simulink model "MultiBody2024bfinal"  (R2024b)
settings: Solver=ode45  StartTime=0.0  StopTime=5  FixedStep=0.001  RelTol=1e-3  AbsTol=1e-3  EnableMultiTasking=on
InitFcn:
  | contact_damping = 1e4;
  | contact_stiffness = 1e6;
values from neighbouring files (symbols this model uses):
  Angle = [30 30 0]    [main_SuperTwistingSMC2.m]
  Height = -(1.9 + i)    (= -5.9)    [main_SuperTwistingSMC2.m]
  i = 4    [main_SuperTwistingSMC2.m]
  nt = n_t(i)    [main_SuperTwistingSMC2.m]
  TM = TMM(i)    [main_SuperTwistingSMC2.m]
  TotalWeight = TotalWeightmb(i)    [main_SuperTwistingSMC2.m]
undefined symbols (not defined in the file or in its folder): X, Y, Z
libraries: sm_lib x207, nesl_utility x73, sharedtransform x6, simulink_extras x4
(part 1 of 7)
settings Model: Creator=anaderi  LastModifiedBy=a.naderi
settings SolverCC: AutoScaleAbsTol=off  MaxZcPerStep=1
settings DataIOCC: LimitDataPoints=on  MaxDataPoints=10000
settings OptimizationCC: ReuseModelBlockBuffer=off  LifeSpan=inf
settings DebuggingCC: UnconnectedInputMsg=warning  UnconnectedOutputMsg=warning  UnconnectedLineMsg=warning  AllowSymbolicDim=off  SFUnexpectedBacktrackingDiag=warning  SFNoUnconditionalDefaultTransitionDiag=warning  SFExecutionAtInitializationDiag=none  ArithmeticOperatorsInVariantConditions=warning
settings ModelReferenceCC: EnableRefExpFcnMdlSchedulingChecks=on
settings SFSimCC: SimUseLocalCustomCode=off  CustomCodeUndefinedFunction=UseInterfaceOnly
settings RTWCC: RTWUseLocalCustomCode=off  GPUComputeCapability=3.5  DLArmComputeVersion=19.05
settings CodeAppCC: StateflowObjectComments=on
settings GRTTargetCC: TargetLangStandard=C89/C90 (ANSI)
settings ConfigComp: CovMetricSettings=dw  CovSaveCumulativeToWorkspaceVar=on  CovSaveSingleToWorkspaceVar=on  CovExternalEMLEnable=off  CovSFcnEnable=off
settings SimscapeCC: SimscapeLogType=all  SimscapeLogSimulationStatistics=on  SimscapeLogDataHistory=10000
settings ExplorerConfigSet: InternalSimMechanicsExplorerSettings="<ExplorerConfiguration><canonicalview>planar_xy</canonicalview><AnimationSetting><BasePlaybackSpeed>1.0</BasePlaybackSpeed><PlaybackSpeedFactor>1.0</PlaybackSpeedFactor></AnimationSetting><TilePanel><TileInfo><Tiles Columns=\"1\" Count=\"1\" Rows=\"1\"><Column Weight=\"1\"/><Row Weight=\"1\"/><Tile Height=\"1\" Width=\"1\" X=\"0\" Y=\"0\"/></Tiles></TileInfo><SceneInfo><SceneViewer><BGColor><R>1</R><G>1</G><B>1</B></BGColor><Camera><DoPerspective>off</DoPerspective><Position><X>-7.52643127180251614</X><Y>2.63618993258771184</Y><Z>6.23451341637808731</Z></Position><Center><X>-0.112830566017771972</X><Y>-0.116652157255869859</Y><Z>3.01253102664829608</Z></Center><Up><X>0.102173989792677611</X><Y>-0.627892603106608771</Y><Z>0.771564225955203575</Z></Up><ViewLimDist>1</ViewLimDist><YLim>1.72776258426052953</YLim><XLim>2.67975369164909827</XLim></Camera></SceneViewer></SceneInfo></TilePanel><MechEditorPanel><Cameras/><GfxPanelCameraMap/><VideoCreator><PlaybackSpeedRatio>1.0</PlaybackSpeedRatio><FrameRate>30</FrameRate><VideoFormat>Motion JPEG AVI</VideoFormat><FrameSize>auto</FrameSize></VideoCreator></MechEditorPanel></ExplorerConfiguration>"

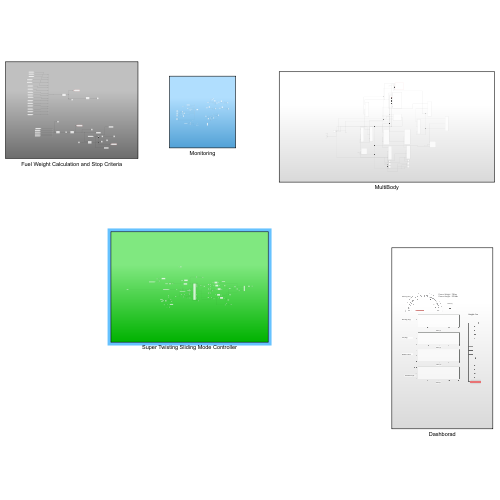
[thumbnail: Simulink's stored preview of the top-level diagram]
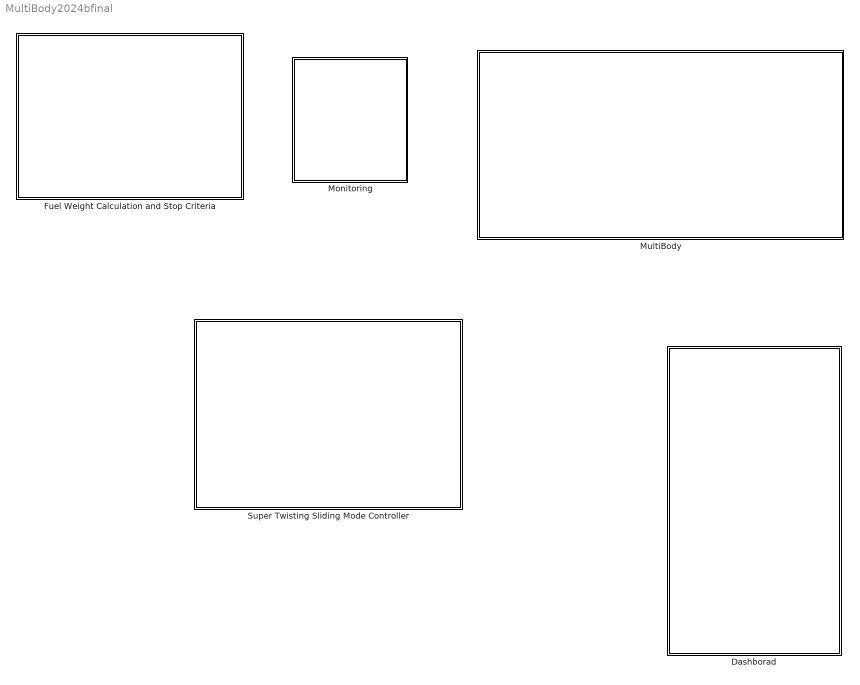
== system MultiBody2024bfinal ==
  Dashborad : Subsystem
  Fuel Weight Calculation and Stop Criteria : Subsystem
  Monitoring : Subsystem
  MultiBody : Subsystem
  Super Twisting Sliding Mode Controller : Subsystem

== system MultiBody2024bfinal/Dashborad ==
  note: Person Weight : 75 kg
      | Person Height : 170 cm
  note: Height: 3m
  note: Velocity (m/s)
  note: Time (s)
  note: Time (s)
  note: Bending (deg)
  note: Tilt (deg)
  note: Time (s)
  note: Rotation (deg)
  note: Time (s)
  note: Time (s)
  note: Disturbance (N)
  Dashboard Scope : DashboardScope  TimeSpan=2  Ymin=-50  Ymax=40  LegendPosition=InsideRight  ScaleAtStop=off
  Dashboard Scope1 : DashboardScope  TimeSpan=2  Ymin=-40  Ymax=30  LegendPosition=InsideRight  ScaleAtStop=off
  Dashboard Scope2 : DashboardScope  TimeSpan=2  Ymin=-180  Ymax=180  LegendPosition=InsideRight  ScaleAtStop=off
  Dashboard Scope3 : DashboardScope  TimeSpan=2  Ymin=0  Ymax=1100  LegendPosition=InsideRight  ScaleAtStop=off
  Display : DisplayBlock  LabelPosition=Hide  Transparency=1  Layout=Fill available space
  Half Gauge : SemiCircularGaugeBlock  LabelPosition=Hide  ScaleMax=12
  Vertical Gauge : CustomWebBlock  LabelPosition=Hide  ShowInitialText=on  Configuration="{\"components\":[{\"name\":\"LinearScaleComponent\",\"settings\":{\"bounds\":{\"max\":3,\"min\":0,\"tickInterval\":\"auto\"},\"internalTickHeightScaleFactor\":0.5,\"labelColor\":[0,0,0],\"labelFont\":{\"font\":\"Arial\",\"fontSize\":12},\"labelOffset\":0.05,\"labelTransparency\":1,\"needleImage\":{\"size\":[21,75],\"src\":\"data:image\\/svg+xml;base64,PHN2ZyB4bWxucz0iaHR0cDovL3d3dy53My5vcmcvMjAwMC9zdmciIHhtbG5zOnhsaW5rPSJodHRwOi8vd3d3LnczLm9yZy8xOTk5L3hsaW5rIiB2aWV3Qm94PSIwIDAgMjEgNzUiPjxkZWZzPjxzdHlsZT4uY2xzLTF7ZmlsbDpub25lO30uY2xzLTJ7aXNvbGF0aW9uOmlzb2xhdGU7fS5jbHMtM3tjbGlwLXBhdGg6dXJsKCNjbGlwLXBhdGgpO30uY2xzLTR7b3BhY2l0eTowLjM7bWl4LWJsZW5kLW1vZGU6bXVsdGlwbHk7fS5jbHMtNXtmaWxsOiNlYjI2Mjk7fTwvc3R5bGU+PGNsaXBQYXRoIGlkPSJjbGlwLXBhdGgiIHRyYW5zZm9y ...(+1928 chars)\",\"srcOrientation\":\"horizontal\"},\"needleOffset\":[0.007413509060955519,0],\"needleSize\":{\"height\":0.11955094537815127,\"width\":0.7589285714285714},\"position\":[0.015811846038863975,0.0696875,0.79984375,0.9641489162929746],\"referencePoint\":\"auto\",\"scaleColors\":[],\"scaleColorsSize\":0.2,\"scaleDirection\":\"BT\",\"showLabels\":1,\"showMinorTicks\":0,\"showSpanLine\":1,\"showTicks\":1,\"tickColor\":[0,0,0],\"tickTransparency\":1,\"valueBarColor\":[23,89,176],\"valueBarOffset\":-1,\"valueBarSize\":0,\"valueBarTransparency\":1}},{\"name\":\"BackgroundImageComponent\",\"settings\":{\"image\":{\"size\":[380,101],\"src\":\"data:image\\/svg+xml;base64,PHN2ZyBpZD0iZnJhbWUiIHhtbG5zPSJodHRwOi8vd3d3LnczLm9yZy8yMDAwL3N2ZyIgeG1sbnM6eGxpbms9Imh0dHA6Ly93d3cudzMub3JnLzE5OTkveGxpbmsiIHZpZXdCb3g9IjAgMCAzODAgMTAxIj48ZGVmcz48c3R5bGU+LmNscy0xe2ZpbGw6IzAwMmI0Mjt9LmNscy0ye2ZpbGw6IzQyNzA4Mjt9LmNscy0ze2ZpbGw6dXJsKCNyYWRpYWwtZ3JhZGllbnQpO308L3N0eWxlPjxyYWRpYWxHcmFkaWVudCBpZD0icmFkaWFsLWdyYWRpZW50IiBjeD0iMTkwIiBjeT0iNTAuNSIgcj0iMjY5LjIxIiBncmFkaWVudFVuaXRzPSJ1c2VyU3BhY2VPblVzZSI+PHN0b3Agb2Zmc2V0PSIwLjAxIiBzdG9wLWNvbG9yPSIjM2U0ZjU4Ii8+PHN0b3Agb2Zmc2V0PSIwLjA2IiBzdG9wLWNvbG9yPSIjNDQ1NzYxIi8+PHN0b3Agb2Zmc2V0PSIwLjE1IiBzdG9wLWNvbG9yPSIjNTU2YTc2Ii8+PHN0b3Agb2Zmc2V0PSIwLjI1IiBzdG9wLWNvbG9yPSIjNmQ4ODk1Ii8+PHN0b3Agb2Zmc2V0PSIwLjM4IiBzdG9wLWNvbG9yPSIjOGZiMmMzIi8+PHN0b3Agb2Zmc2V0PSIwLjUyIiBzdG9wLWNvbG9yPSIjYjZlNGZhIi8+PHN0b3Agb2Zmc2V0PSIxIiBzdG9wLWNvbG9yPSIjMTU0NjU3Ii8+PC9yYWRpYWxHcmFkaWVudD48L2RlZnM+PGcgaWQ9IkxheWVyXzIiIGRhdGEtbmFtZT0iTGF5ZXIgMiI+PGcgaWQ9IkxheWVyXzEtMiIgZGF0YS1uYW1lPSJMYXllciAxLTIiPjxyZWN0IGlkPSJyZWN0MTAzNiIgY2xhc3M9ImNscy0xIiB4PSIxMSIgeT0iMTEiIHdpZHRoPSIzNTgiIGhlaWdodD0iNzkiLz48cGF0aCBpZD0icGF0aDEwMzgiIGNsYXNzPSJjbHMtMiIgZD0iTTgsOFY5M0gzNzJWOFpNMzY5LDkwSDExVjExSDM2OVoiLz48cGF0aCBpZD0icGF0aDEwNDAiIGNsYXNzPSJjbHMtMyIgZD0iTTAsMFYxMDFIMzgwVjBaTTM3Miw5M0g4VjhIMzcyWiIvPjwvZz48L2c+PC9zdmc+\",\"srcOrientation\":\"horizontal\"},\"position\":[0,0,1,1],\"scaleMode\":\"0\"}},{\"name\":\"ForegroundImageComponent\",\"settings\":{\"image\":{\"size\":[0,0],\"src\":\"default\",\"srcOrientation\":[]},\"isForeground\":1,\"position\":[0,0,1,1],\"scaleMode\":\"0\"}}],\"settings\":{\"BindingType\":\"signal\",\"backgroundColor\":[0,0,0,\"1\"],\"backgroundOffset\":0,\"backgroundOpacity\":0,\"fixedAspectRatio\":\"off\",\"orientation\":\"vertical\",\"showBackgroundColor\":false,\"value\":0,\"version\":\"R2022b\"},\"type\":\"LinearGauge\"}"  CustomBackgroundColor="{\"color\":[1,1,1],\"show\":true}"

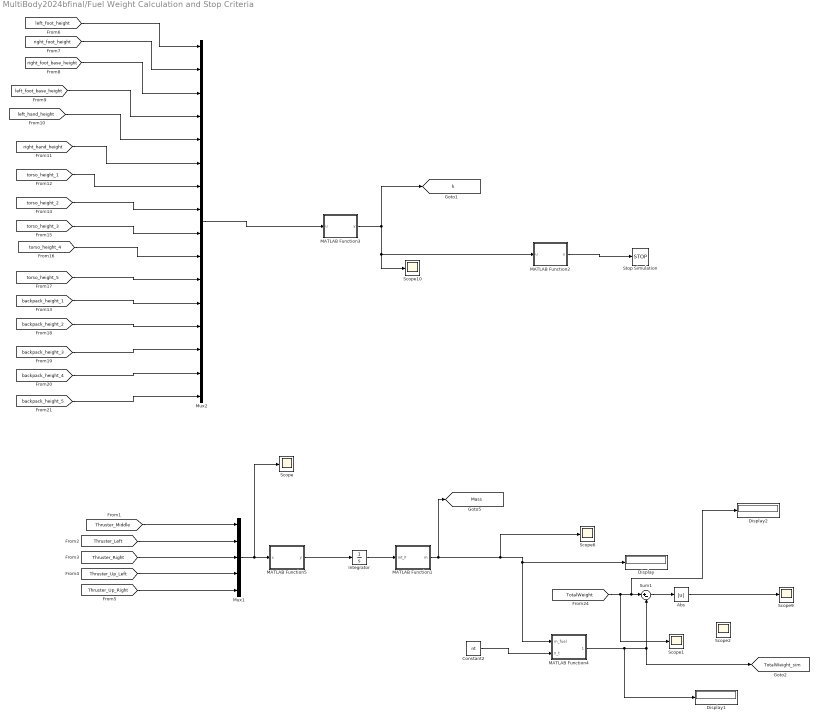
== system MultiBody2024bfinal/Fuel Weight Calculation and Stop Criteria ==
  Abs : Abs  SaturateOnIntegerOverflow=off
  Constant2 : Constant  Value=nt
  Display : Display
  Display1 : Display
  Display2 : Display
  Integrator : Integrator
  MATLAB Function1 : MATLAB Function  TreatAsAtomicUnit=on
  MATLAB Function2 : MATLAB Function  TreatAsAtomicUnit=on
  MATLAB Function3 : MATLAB Function  TreatAsAtomicUnit=on
  MATLAB Function4 : MATLAB Function  TreatAsAtomicUnit=on
  MATLAB Function5 : MATLAB Function  TreatAsAtomicUnit=on
  Mux1 : Mux  Inputs=5
  Mux2 : Mux  Inputs=16
  Scope{,1..2,6,9..10} (6 alike) : Scope
  Stop Simulation : Stop
  Sum1 : Sum  Inputs=|+-
  tag scope: Mass=global, TotalWeight_sim=global, h=global
  wires:
  [torso_height_2] -> Mux2/8
  MATLAB Function4/1(m_total) -> Display1/1, Sum1/2, [TotalWeight_sim]
  MATLAB Function1/1(m) -> Scope6/1, MATLAB Function4/1(m_fuel), Display/1, [Mass]
  MATLAB Function5/1(y) -> Integrator/1
  [backpack_height_2] -> Mux2/13
  [right_foot_height] -> Mux2/2
  [backpack_height_1] -> Mux2/12
  [left_foot_base_height] -> Mux2/4
  [backpack_height_4] -> Mux2/15
  Sum1/1 -> Abs/1
  Mux1/1 -> Scope/1, MATLAB Function5/1(x)
  Mux2/1 -> MATLAB Function3/1(u)
  [right_hand_height] -> Mux2/6
  [backpack_height_5] -> Mux2/16
  [torso_height_3] -> Mux2/9
  [torso_height_5] -> Mux2/11
  [Thruster_Right] -> Mux1/3
  [left_hand_height] -> Mux2/5
  [torso_height_4] -> Mux2/10
  [backpack_height_3] -> Mux2/14
  MATLAB Function2/1(y) -> Stop Simulation/1
  [left_foot_height] -> Mux2/1
  [Thruster_Up_Left] -> Mux1/4
  MATLAB Function3/1(y) -> MATLAB Function2/1(u), Scope10/1, [h]
  [Thruster_Middle] -> Mux1/1
  [right_foot_base_height] -> Mux2/3
  [torso_height_1] -> Mux2/7
  [Thruster_Up_Right] -> Mux1/5
  Abs/1 -> Scope9/1
  [Thruster_Left] -> Mux1/2
  Constant2/1 -> MATLAB Function4/2(n_t)
  Integrator/1 -> MATLAB Function1/1(int_F)
  [TotalWeight] -> Scope1/1, Display2/1, Sum1/1

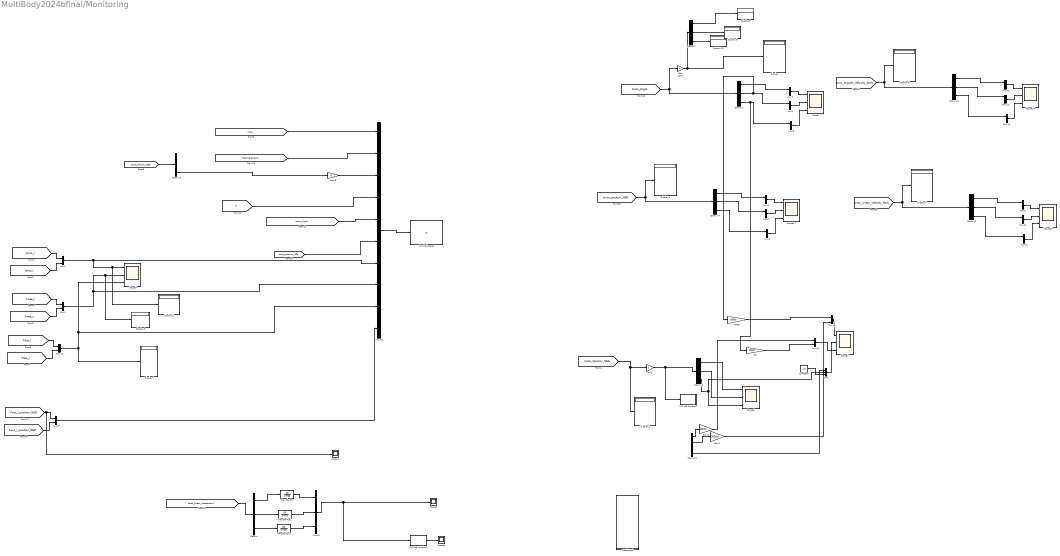
== system MultiBody2024bfinal/Monitoring ==
  Constant : Constant  Value=4.8
  Dashborad : Subsystem
  Demux{,1..4,6..8} (8 alike) : Demux  Outputs=3
  Demux5 : Demux
  Display{,1..10} (11 alike) : Display
  Gain : Gain  Gain=180/pi
  Gain1 : Gain  Gain=180/pi
  Gain6 : Gain  Gain=180/pi
  Gain8 : Gain  Gain=-1
  MATLAB Function : MATLAB Function  TreatAsAtomicUnit=on
  MATLAB Function1 : MATLAB Function  TreatAsAtomicUnit=on
  Mux : Mux  Inputs=3
  Mux{1..15,17,19..20} (18 alike) : Mux  Inputs=2
  Mux16 : Mux  Inputs=10
  Mux18 : Mux  Inputs=3
  Phi : Gain  Gain=180/pi
  Phi2 : Gain
  Scope{,1..3,17,19..20} (7 alike) : Scope  NumInputPorts=3
  Scope4 : Scope
  Scope5 : Scope
  Scope6 : Scope
  Theta : Gain  Gain=180/pi
  To Workspace : ToWorkspace  VariableName=x  SampleTime=-1
      settings: Save2DSignal=2-D array (concatenate along first dimension)
  Transfer Fcn : TransferFcn  Numerator=[50]  Denominator=[1 50]
  Transfer Fcn1 : TransferFcn  Numerator=[50]  Denominator=[1 50]
  Transfer Fcn2 : TransferFcn  Numerator=[50]  Denominator=[1 50]
  wires:
  [torso_Angle] -> Demux2/1, Gain/1
  [torso_position_NED] -> Demux4/1, Display2/1
  Mux7/1 -> Scope17/2
  Demux4/2 -> Mux7/1
  [torso_Linear_Velocity_Body] -> Display4/1, Demux6/1
  Mux4/1 -> Scope/2
  Demux6/1 -> Mux9/1
  Demux2/2 -> Theta/1, Mux4/1
  [torso_Angular_Velocity_Body] -> Demux8/1, Display6/1
  Demux6/2 -> Mux10/1
  Mux10/1 -> Scope19/2
  Mux6/1 -> Scope17/1
  Mux9/1 -> Scope19/1
  Mux11/1 -> Scope19/3
  Mux12/1 -> Scope20/2
  Mux8/1 -> Scope17/3
  Mux14/1 -> Scope20/1
  Mux5/1 -> Scope/3
  Mux3/1 -> Scope/1
  Demux8/1 -> Mux14/1
  Demux2/3 -> Phi/1, Mux5/1
  Demux4/1 -> Mux6/1
  Demux2/1 -> Mux3/1
  Demux8/3 -> Mux13/1
  Demux8/2 -> Mux12/1
  Demux6/3 -> Mux11/1
  Mux13/1 -> Scope20/3
  Demux4/3 -> Mux8/1
  Theta/1 -> Mux19/1
  [torso_Velocity_NED] -> Display1/1, Phi2/1
  Demux1/3 -> Mux/2, Scope2/3
  Phi/1 -> Mux20/2
  Gain/1 -> Demux7/1, Display/1
  Constant/1 -> Mux/3
  Mux/1 -> Scope1/2
  Demux1/1 -> Scope2/1
  Demux1/2 -> Scope2/2
  Phi2/1 -> Demux1/1, MATLAB Function/1(u)
  [torso_r] -> Mux1/1
  [torso_l] -> Mux1/2
  [knee_r] -> Mux2/2
  [knee_l] -> Mux2/1
  [Tibia_l] -> Mux15/1
  [Tibia_r] -> Mux15/2
  Mux2/1 -> Mux16/8, Display5/1, Scope3/2
  [torso_Velocity_NED] -> Demux3/1
  Demux3/3 -> Gain8/1
  [torso_Angle] -> Mux16/5
  Mux16/1 -> To Workspace/1
  [TotalWeight_sim] -> Mux16/2
  [torso_position_NED] -> Mux16/6
  Gain8/1 -> Mux16/3
  [h] -> Mux16/4
  [Mass] -> Mux16/1
  Mux1/1 -> Mux16/7, Display3/1, Scope3/1
  Mux15/1 -> Mux16/9, Scope3/3, Display7/1
  [Foot_r_position_NED] -> Mux17/2
  [Foot_l_position_NED] -> Scope4/1, Mux17/1
  Mux17/1 -> Mux16/10
  Mux18/1 -> MATLAB Function1/1(u), Scope5/1
  [torso_Linear_Acceleration] -> Demux/1
  Demux/1 -> Transfer Fcn/1
  Transfer Fcn/1 -> Mux18/1
  Demux/2 -> Transfer Fcn1/1
  Transfer Fcn1/1 -> Mux18/2
  Demux/3 -> Transfer Fcn2/1
  Transfer Fcn2/1 -> Mux18/3
  MATLAB Function1/1(y) -> Scope6/1
  Demux5/2 -> Gain1/1
  ? -> Demux5/1
  Demux5/1 -> Gain6/1
  Gain1/1 -> Mux19/2
  Mux19/1 -> Scope1/1
  Gain6/1 -> Mux20/1
  Mux20/1 -> Scope1/3
  Demux5/4 -> Mux/1
  Demux7/1 -> Display8/1
  Demux7/2 -> Display9/1
  Demux7/3 -> Display10/1

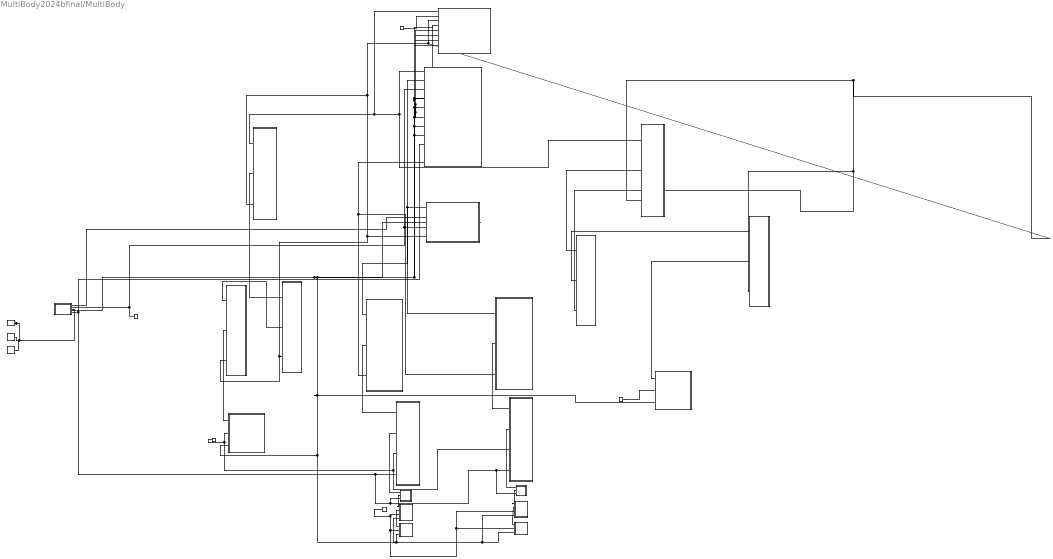
== system MultiBody2024bfinal/MultiBody ==
  Connection Label{1..5} (5 alike) : ConnectionLabel  Label=Ground
  Femur_r : Subsystem
      mask Display: image('$imagefile');
  Femur_r1 : Subsystem
      mask Display: image('$imagefile'); % Use "Edit Image" on toolstrip to change.
  Femur_r10 : Subsystem
      mask Display: image('$imagefile'); % Use "Edit Image" on toolstrip to change.
  Femur_r11 : Subsystem
      mask Display: image('$imagefile'); % Use "Edit Image" on toolstrip to change.
  Femur_r12 : Subsystem
      mask Display: image('$imagefile'); % Use "Edit Image" on toolstrip to change.
  Femur_r13 : Subsystem
      mask Display: image('$imagefile'); % Use "Edit Image" on toolstrip to change.
  Femur_r14 : Subsystem
      mask Display: image('$imagefile'); % Use "Edit Image" on toolstrip to change.
  Femur_r15 : Subsystem
      mask Display: image('$imagefile'); % Use "Edit Image" on toolstrip to change.
  Femur_r2 : Subsystem
      mask Display: image('$imagefile'); % Use "Edit Image" on toolstrip to change.
  Femur_r3 : Subsystem
      mask Display: image('$imagefile'); % Use "Edit Image" on toolstrip to change.
  Femur_r4 : Subsystem
      mask Display: image('$imagefile'); % Use "Edit Image" on toolstrip to change.
  Femur_r5 : Subsystem
      mask Display: image('$imagefile'); % Use "Edit Image" on toolstrip to change.
  Femur_r6 : Subsystem
      mask Display: image('$imagefile'); % Use "Edit Image" on toolstrip to change.
  Femur_r7 : Subsystem
      mask Display: image('$imagefile'); % Use "Edit Image" on toolstrip to change.
  Femur_r8 : Subsystem
      mask Display: image('$imagefile'); % Use "Edit Image" on toolstrip to change.
  Femur_r9 : Subsystem
      mask Display: image('$imagefile'); % Use "Edit Image" on toolstrip to change.
  Grpund : Subsystem
  Mechanism Configuration : sm_lib/Utilities/Mechanism Configuration  UniformGravity=Constant  GravityVector=[0 0 -9.80665]  GravityVectorUnits=m/s^2  LinearizationDelta=0.001  JointModeTransitionNonlinearIterations=2
  Pelvos : Subsystem
      mask Display: image('$imagefile'); % Use "Edit Image" on toolstrip to change.
  Solver Configuration : nesl_utility/Solver Configuration  PhysicalDomain=network_engine_domain  SubClassName=solver  LeftPortType=input  RightPortType=generic  Tones=[]  Harmonics=[]  SimulateNoise=off  Profile=off  UseLocalSampling=off  EnableSwitchedLinearOptims=on  FrequencyDomain=off  UseCCode=off  RelTol=0.001  AbsTol=1e-06  MinStep=1e-09  ToWorkspace=off  RevertToSquareIcSolve=off  NumHomotopyIterations=100  PhasorMode=off  PhasorModeNumHarmonics=1  ConsistencySolver=NEWTON_FTOL  IndexReductionMethod=DerivativeReplacement  DoDC=off  ResidualTolerance=1e-09  ConsistencyTolSource=GLOBAL  ConsistencyAbsTol=0.001  ConsistencyRelTol=0.001  ConsistencyTolFactor=0.001  UseLocalSolver=off  LocalSolverChoice=NE_BACKWARD_EULER_ADVANCER  ResolveIndetEquations=on  FunctionEvalNumThread=1  LocalSolverSampleTime=0.001  DoFixedCost=off  MaxNonlinIter=3  MaxModeIter=2  ComputeImpulses=off  ImpulseIterations=2  LinearAlgebra=Sparse  LinearAlgebraNumThread=0  EquationFormulation=NE_TIME_EF  DelaysMemoryBudget=1024  AutomaticFiltering=on  FilteringTimeConstant=0.001  PartitionStorageMethod=AS_NEEDED  PartitionMemoryBudget=1024  PartitionMethod=FAST  MultibodyUseLocalSolver=off  MultibodyLocalSolverChoice=ODE1  MultibodyLocalSolverSampleTime=0.001
  Tibia _r : Subsystem
      mask Display: image('$imagefile'); % Use "Edit Image" on toolstrip to change.
  Tibia _r1 : Subsystem
      mask Display: image('$imagefile'); % Use "Edit Image" on toolstrip to change.
  Torso : Subsystem
      mask Display: image('$imagefile'); % Use "Edit Image" on toolstrip to change.
  Truster Unit : Subsystem
      mask Display: image('$imagefile'); % Use "Edit Image" on toolstrip to change.
  World Frame : sm_lib/Frames and Transforms/World Frame
  connections:
  Femur_r15/LConn3 -- Femur_r14/LConn4 -- Femur_r11/LConn4 -- Femur_r6/LConn3 -- Femur_r9/LConn3 -- Grpund/RConn4 -- Truster Unit/LConn8 -- Truster Unit/LConn7 -- Truster Unit/LConn6 -- Truster Unit/LConn5 -- Truster Unit/LConn4 -- Torso/LConn4 -- Torso/LConn5 -- Torso/LConn6 -- Torso/LConn7 -- Torso/LConn8 -- Pelvos/RConn1 -- Femur_r12/LConn3
  Pelvos/LConn1 -- Femur_r/LConn1 -- Femur_r1/LConn1 -- Torso/LConn2
  Femur_r12/LConn1 -- Femur_r11/LConn2
  Connection Label5/LConn1 -- Femur_r9/LConn2
  Connection Label2/LConn1 -- Femur_r15/LConn2 -- Femur_r14/LConn3 -- Femur_r12/LConn2 -- Femur_r11/LConn3
  Connection Label4/LConn1 -- Tibia _r1/LConn3 -- Tibia _r/LConn3 -- Femur_r6/LConn2
  Tibia _r/LConn2 -- Femur_r10/LConn1
  Femur_r14/LConn1 -- Femur_r13/LConn2
  Truster Unit/LConn1 -- Femur_r3/LConn1 -- Femur_r2/LConn1 -- Torso/LConn1
  Femur_r4/LConn2 -- Femur_r5/LConn1
  Connection Label1/LConn1 -- Torso/LConn3 -- Pelvos/LConn3 -- Grpund/RConn2
  Femur_r8/LConn1 -- Femur_r7/LConn2
  Pelvos/LConn2 -- Grpund/RConn1
  Femur_r1/LConn2 -- Tibia _r1/LConn1
  Femur_r4/LConn1 -- Femur_r3/LConn2
  Femur_r8/LConn2 -- Femur_r9/LConn1
  Femur_r15/LConn1 -- Femur_r14/LConn2
  Femur_r7/LConn1 -- Femur_r2/LConn2
  Femur_r13/LConn1 -- Tibia _r1/LConn2
  Femur_r/LConn2 -- Tibia _r/LConn1
  Connection Label3/LConn1 -- Truster Unit/LConn2
  Femur_r11/LConn1 -- Femur_r10/LConn2
  Solver Configuration/RConn1 -- Grpund/RConn3 -- World Frame/RConn1 -- Mechanism Configuration/RConn1
  Femur_r5/LConn2 -- Femur_r6/LConn1
  Pelvos/LConn4 -- Femur_r3/LConn3 -- Femur_r2/LConn3 -- Femur_r7/LConn3 -- Femur_r8/LConn3 -- Truster Unit/LConn3 -- Femur_r5/LConn3 -- Femur_r4/LConn3
  Torso/LConn9 -- Femur_r10/LConn3 -- Femur_r13/LConn3 -- Tibia _r1/LConn4 -- Tibia _r/LConn4 -- Grpund/RConn5
  Torso/LConn11 -- Femur_r1/LConn3 -- Femur_r/LConn3

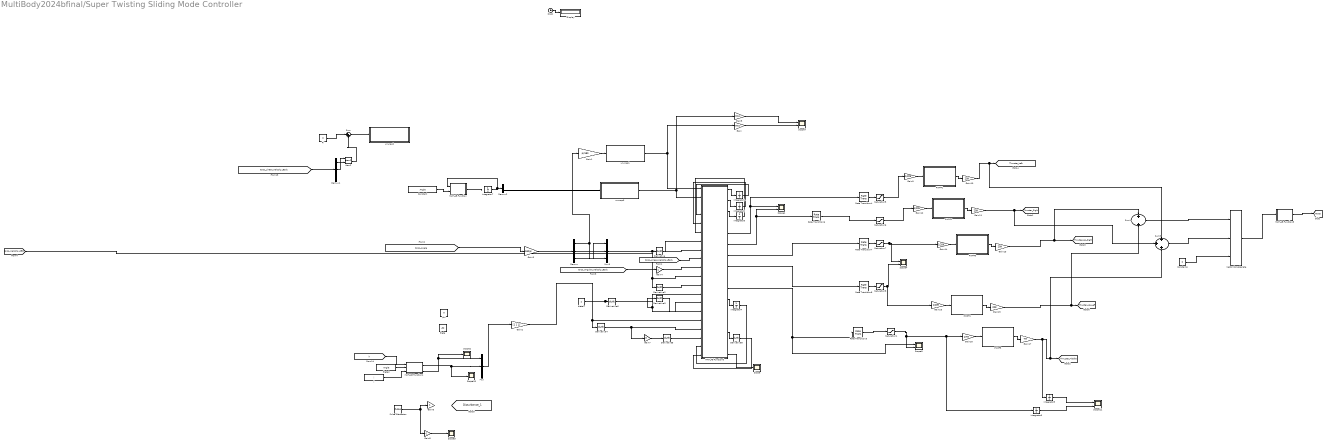
== system MultiBody2024bfinal/Super Twisting Sliding Mode Controller ==
  Atan2 : Trigonometry  Operator=atan2
  Clock : Clock
  Constant : Constant  Value=Angle
  Constant4 : Constant  Value=0
  Demux : Demux  Outputs=3
  Demux1 : Demux  Outputs=3
  Demux2 : Demux  Outputs=3
  Derivative{,2..6,8} (7 alike) : Derivative
  Display : Display
  Gain : Gain  Gain=180/pi
  Gain1 : Gain  Gain=pi/180
  Gain{10..11,13,15} (4 alike) : Gain  Gain=209
  Gain{9,12,14,16} (4 alike) : Gain  Gain=1/209
  Gain17 : Gain  Gain=TM
  Gain18 : Gain  Gain=1/TM
  Gain2 : Gain  Gain=[1 1 1]'
  Gain3 : Gain  Gain=180/pi
  Gain4 : Gain
  Gain5 : Gain  Gain=180/pi
  Gain6 : Gain
  Gain7 : Gain  Gain=0
  Gain8 : Gain  Gain=-1
  Integrator{1..6} (6 alike) : Integrator
  Integrator7 : Integrator  InitialCondition=[0 0 Angle(3)*pi/180]'
  MATLAB Function : MATLAB Function  TreatAsAtomicUnit=on
  MATLAB Function1 : MATLAB Function  TreatAsAtomicUnit=on
  MATLAB Function6 : MATLAB Function  TreatAsAtomicUnit=on
  MATLAB Function8 : MATLAB Function  TreatAsAtomicUnit=on
  Mux : Mux  Inputs=3
  Mux3 : Mux  Inputs=3
  PWPF1 : Subsystem  mask{Um=1, Uon=0.1, Uoff=0.01, Km=50, Tm=0.1}
      mask prompts: Um "U"; Km "Km(Filter Gain)"; Tm "Tm(Filter Time Constant)"
  PWPF2 : Subsystem  mask{Um=1, Uon=0.1, Uoff=0.01, Km=50, Tm=0.1}
      mask prompts: Um "U"; Km "Km(Filter Gain)"; Tm "Tm(Filter Time Constant)"
  PWPF3 : Subsystem  mask{Um=1, Uon=0.1, Uoff=0.01, Km=50, Tm=0.1}
      mask prompts: Um "U"; Km "Km(Filter Gain)"; Tm "Tm(Filter Time Constant)"
  PWPF4 : Subsystem  mask{Um=1, Uon=0.1, Uoff=0.01, Km=50, Tm=0.1}
      mask prompts: Um "U"; Km "Km(Filter Gain)"; Tm "Tm(Filter Time Constant)"
  PWPF5 : Subsystem  mask{Um=1, Uon=0.1, Uoff=0.01, Km=100, Tm=0.1}
      mask prompts: Um "U"; Km "Km(Filter Gain)"; Tm "Tm(Filter Time Constant)"
  Pi : Constant  Value=0  OutDataTypeStr=Inherit: Inherit via back propagation
  Pulse Generator : DiscretePulseGenerator  PulseType=Time based  Amplitude=-1000  Period=5
  Rate Transition{3..4,6..8} (5 alike) : RateTransition
  Saturation1 : Saturate  UpperLimit=TM  LowerLimit=0
  Saturation5 : Saturate  UpperLimit=209  LowerLimit=0
  Saturation6 : Saturate  UpperLimit=209  LowerLimit=0
  Saturation7 : Saturate  UpperLimit=209  LowerLimit=-209
  Saturation8 : Saturate  UpperLimit=209  LowerLimit=-209
  Scope{,2..3,10} (4 alike) : Scope
  Scope{1,4..5,7,11} (5 alike) : Scope  NumInputPorts=2
  Sum : Sum  Inputs=|++
  Sum1 : Sum
  Sum3 : Sum  Inputs=+++
  Vector Concatenate : Concatenate  NumInputs=3
  i : Constant  Value=i
  phi : Constant  Value=0
  theta : Constant  Value=-30
  theta1 : Constant  Value=2
  theta2 : Constant  Value=Angle
  unwrap1 : Subsystem
  unwrap2 : Subsystem
  unwrap3 : Subsystem
  tag scope: Disturbance_1=global, Force=global, Thruster_Left=global, Thruster_Middle=global, Thruster_Right=global, Thruster_Up_Left=global, Thruster_Up_Right=global
  wires:
  Demux1/1 -> Atan2/2
  Demux1/2 -> Atan2/1
  [torso_Angular_Velocity_Body] -> Gain4/1
  [torso_Angle] -> Gain3/1
  MATLAB Function6/1(dz1) -> Integrator1/1
  Mux3/1 -> MATLAB Function6/7(eta), Derivative/1
  Gain3/1 -> Demux/1
  Gain1/1 -> unwrap1/1(input_angle)
  Mux/1 -> Gain2/1
  Demux/2 -> Mux3/2
  Demux/1 -> Mux3/3, Gain1/1
  Demux/3 -> Mux3/1
  MATLAB Function6/3(dz3) -> Integrator3/1
  MATLAB Function6/2(dz2) -> Integrator2/1
  theta1/1 -> MATLAB Function6/13(v_d), Derivative6/1
  Gain2/1 -> Derivative4/1, MATLAB Function6/16("eta_d ")
  [torso_Velocity_NED] -> Derivative2/1, MATLAB Function6/11(v_NED)
  Derivative6/1 -> MATLAB Function6/14(dv_d), Derivative3/1
  MATLAB Function6/5(T_Left) -> Rate Transition4/1, Scope1/1
  Rate Transition7/1 -> Saturation7/1
  Derivative/1 -> MATLAB Function6/8(deta)
  Derivative8/1 -> MATLAB Function6/20(de4)
  [torso_Linear_Velocity_Body] -> MATLAB Function6/9(v1)
  Gain4/1 -> MATLAB Function6/10(v2)
  Derivative2/1 -> MATLAB Function6/12(dv_NED)
  Derivative3/1 -> MATLAB Function6/15(ddv_d)
  Derivative5/1 -> MATLAB Function6/18(ddeta_d)
  Rate Transition4/1 -> Saturation5/1
  Gain5/1 -> Scope7/1
  Gain/1 -> Scope7/2
  MATLAB Function6/7(T_Up_Right) -> Rate Transition7/1
  MATLAB Function6/6(T_Right) -> Scope1/2, Rate Transition6/1
  MATLAB Function6/8(T_Up_Left) -> Rate Transition8/1
  MATLAB Function6/11(dz4) -> Integrator4/1
  MATLAB Function6/10(T_Middle) -> Scope5/1, Rate Transition3/1
  MATLAB Function6/14(e4) -> Derivative8/1
  Rate Transition3/1 -> Saturation1/1
  Integrator2/1 -> MATLAB Function6/5(z2)
  Rate Transition8/1 -> Saturation8/1
  Integrator1/1 -> MATLAB Function6/4(z1)
  Rate Transition6/1 -> Saturation6/1
  PWPF1/1(Thrust) -> Gain10/1
  Integrator3/1 -> MATLAB Function6/6(z3)
  Integrator4/1 -> MATLAB Function6/19(z4)
  Sum/1 -> unwrap2/1(input_angle)
  Atan2/1 -> Sum/2
  Pi/1 -> Sum/1
  Saturation7/1 -> Gain14/1, Scope4/1
  Gain9/1 -> PWPF1/1(In1)
  Gain10/1 -> Sum3/1, [Thruster_Left]
  Saturation5/1 -> Gain9/1
  Gain12/1 -> PWPF2/1(In1)
  PWPF2/1(Thrust) -> Gain11/1
  Saturation6/1 -> Gain12/1
  Gain11/1 -> Sum3/2, [Thruster_Right]
  PWPF3/1(Thrust) -> Gain13/1
  Gain14/1 -> PWPF3/1(In1)
  Gain15/1 -> Sum1/2, [Thruster_Up_Left]
  Gain16/1 -> PWPF4/1(In1)
  PWPF4/1(Thrust) -> Gain15/1
  Saturation8/1 -> Gain16/1, Scope4/2
  PWPF5/1(Thrust) -> Gain17/1
  Gain18/1 -> PWPF5/1(In1)
  Gain17/1 -> Integrator5/1, Sum3/3, [Thruster_Middle]
  Integrator6/1 -> Scope11/2
  Saturation1/1 -> Integrator6/1, Gain18/1, Scope5/2
  Integrator5/1 -> Scope11/1
  [torso_Linear_Velocity_Body] -> Demux1/1
  MATLAB Function/1(dX) -> ?
  Integrator7/1 -> Demux2/1, MATLAB Function/1(x)
  MATLAB Function1/1(y1) -> Mux/2, Scope10/1
  [h] -> MATLAB Function1/1(u)
  MATLAB Function6/16(ev) -> Scope/1
  Constant/1 -> MATLAB Function/2(Angle)
  MATLAB Function1/2(y2) -> Mux/1, Scope2/1
  Derivative4/1 -> MATLAB Function6/17(deta_d), Gain7/1
  Gain7/1 -> Derivative5/1
  theta2/1 -> MATLAB Function1/2(Angle)
  unwrap1/1(unwrapped_angle) -> MATLAB Function6/1(psi_m), Gain/1
  Demux2/3 -> unwrap3/1(input_angle)
  Sum1/1 -> Vector Concatenate/1
  Constant4/1 -> Vector Concatenate/3
  Vector Concatenate/1 -> MATLAB Function8/1(u)
  Sum3/1 -> Vector Concatenate/2
  MATLAB Function8/1(y) -> [Force]
  Gain13/1 -> Sum1/1, [Thruster_Up_Right]
  unwrap3/1(unwrapped_angle) -> MATLAB Function6/2(psi_d), Gain5/1
  i/1 -> MATLAB Function1/3(i)
  Pulse Generator/1 -> Gain6/1, Gain8/1
  Clock/1 -> Display/1
  Gain8/1 -> Scope3/1

== system MultiBody2024bfinal/Monitoring/Dashborad ==
  note: Person Weight : 75 kg
      | Person Height : 170 cm
  note: Height: 3m
  note: Velocity(m/s)
  note: Time(s)
  note: Timer(s)
  note: Velocity(m/s)
  Dashboard Scope : DashboardScope  Ymin=0  Ymax=10  LegendPosition=Hide  ScaleAtStop=off
  Display : DisplayBlock  LabelPosition=Hide  Transparency=1  Layout=Fill available space
  Half Gauge : SemiCircularGaugeBlock  LabelPosition=Hide  ScaleMax=10
  Vertical Gauge : CustomWebBlock  Description=Height(m)  LabelPosition=Hide  ShowInitialText=on  Configuration="{\"components\":[{\"name\":\"LinearScaleComponent\",\"settings\":{\"bounds\":{\"max\":5,\"min\":0,\"tickInterval\":\"auto\"},\"internalTickHeightScaleFactor\":0.4,\"labelColor\":[255,255,255],\"labelFont\":{\"font\":\"Arial\",\"fontSize\":12},\"labelOffset\":0.05,\"labelTransparency\":1,\"needleImage\":{\"size\":[21,75],\"src\":\"data:image\\/svg+xml;base64,PHN2ZyB4bWxucz0iaHR0cDovL3d3dy53My5vcmcvMjAwMC9zdmciIHhtbG5zOnhsaW5rPSJodHRwOi8vd3d3LnczLm9yZy8xOTk5L3hsaW5rIiB2aWV3Qm94PSIwIDAgMjEgNzUiPjxkZWZzPjxzdHlsZT4uY2xzLTF7ZmlsbDpub25lO30uY2xzLTJ7aXNvbGF0aW9uOmlzb2xhdGU7fS5jbHMtM3tjbGlwLXBhdGg6dXJsKCNjbGlwLXBhdGgpO30uY2xzLTR7b3BhY2l0eTowLjM7bWl4LWJsZW5kLW1vZGU6bXVsdGlwbHk7fS5jbHMtNXtmaWxsOiNlYjI2Mjk7fTwvc3R5bGU+PGNsaXBQYXRoIGlkPSJjbGlwLXBhdGgiIHRyYW5zZm9y ...(+1928 chars)\",\"srcOrientation\":\"Right\"},\"needleOffset\":[-1.89,0.3],\"needleSize\":{\"height\":0.51,\"width\":4.898},\"position\":[-0.02826037906137184,-0.17999031007751937,0.8373304263565892,1.0712432310469313],\"referencePoint\":\"auto\",\"scaleColors\":[],\"scaleColorsSize\":0.2,\"scaleDirection\":\"BT\",\"showLabels\":true,\"showMinorTicks\":0,\"showSpanLine\":true,\"showTicks\":true,\"tickColor\":[255,255,255],\"tickTransparency\":1,\"valueBarColor\":[0,0,0],\"valueBarOffset\":1,\"valueBarSize\":1,\"valueBarTransparency\":1}},{\"name\":\"BackgroundImageComponent\",\"settings\":{\"image\":{\"size\":[380,101],\"src\":\"data:image\\/svg+xml;base64,PHN2ZyBpZD0iZnJhbWUiIHhtbG5zPSJodHRwOi8vd3d3LnczLm9yZy8yMDAwL3N2ZyIgeG1sbnM6eGxpbms9Imh0dHA6Ly93d3cudzMub3JnLzE5OTkveGxpbmsiIHZpZXdCb3g9IjAgMCAzODAgMTAxIj48ZGVmcz48c3R5bGU+LmNscy0xe2ZpbGw6IzAwMmI0Mjt9LmNscy0ye2ZpbGw6IzQyNzA4Mjt9LmNscy0ze2ZpbGw6dXJsKCNyYWRpYWwtZ3JhZGllbnQpO308L3N0eWxlPjxyYWRpYWxHcmFkaWVudCBpZD0icmFkaWFsLWdyYWRpZW50IiBjeD0iMTkwIiBjeT0iNTAuNSIgcj0iMjY5LjIxIiBncmFkaWVudFVuaXRzPSJ1c2VyU3BhY2VPblVzZSI+PHN0b3Agb2Zmc2V0PSIwLjAxIiBzdG9wLWNvbG9yPSIjM2U0ZjU4Ii8+PHN0b3Agb2Zmc2V0PSIwLjA2IiBzdG9wLWNvbG9yPSIjNDQ1NzYxIi8+PHN0b3Agb2Zmc2V0PSIwLjE1IiBzdG9wLWNvbG9yPSIjNTU2YTc2Ii8+PHN0b3Agb2Zmc2V0PSIwLjI1IiBzdG9wLWNvbG9yPSIjNmQ4ODk1Ii8+PHN0b3Agb2Zmc2V0PSIwLjM4IiBzdG9wLWNvbG9yPSIjOGZiMmMzIi8+PHN0b3Agb2Zmc2V0PSIwLjUyIiBzdG9wLWNvbG9yPSIjYjZlNGZhIi8+PHN0b3Agb2Zmc2V0PSIxIiBzdG9wLWNvbG9yPSIjMTU0NjU3Ii8+PC9yYWRpYWxHcmFkaWVudD48L2RlZnM+PGcgaWQ9IkxheWVyXzIiIGRhdGEtbmFtZT0iTGF5ZXIgMiI+PGcgaWQ9IkxheWVyXzEtMiIgZGF0YS1uYW1lPSJMYXllciAxLTIiPjxyZWN0IGlkPSJyZWN0MTAzNiIgY2xhc3M9ImNscy0xIiB4PSIxMSIgeT0iMTEiIHdpZHRoPSIzNTgiIGhlaWdodD0iNzkiLz48cGF0aCBpZD0icGF0aDEwMzgiIGNsYXNzPSJjbHMtMiIgZD0iTTgsOFY5M0gzNzJWOFpNMzY5LDkwSDExVjExSDM2OVoiLz48cGF0aCBpZD0icGF0aDEwNDAiIGNsYXNzPSJjbHMtMyIgZD0iTTAsMFYxMDFIMzgwVjBaTTM3Miw5M0g4VjhIMzcyWiIvPjwvZz48L2c+PC9zdmc+\",\"srcOrientation\":\"Right\"},\"position\":[0,0,1,1],\"scaleMode\":\"0\"}},{\"name\":\"ForegroundImageComponent\",\"settings\":{\"angle\":0,\"image\":{\"size\":[63,238],\"src\":\"default\",\"srcOrientation\":null},\"isForeground\":1,\"position\":[0,0,1,1],\"scaleMode\":\"0\"}}],\"settings\":{\"BindingType\":\"signal\",\"backgroundColor\":[0,0,0,\"1\"],\"backgroundOffset\":0,\"backgroundOpacity\":1,\"fixedAspectRatio\":\"off\",\"orientation\":\"vertical\",\"showBackgroundColor\":false,\"value\":0,\"version\":\"R2023a\"},\"type\":\"LinearGauge\"}"  CustomBackgroundColor="{\"color\":[0,0.2,0.2],\"show\":true}"
  Vertical Gauge1 : CustomWebBlock  LabelPosition=Hide  ShowInitialText=on  Configuration="{\"components\":[{\"name\":\"LinearScaleComponent\",\"settings\":{\"bounds\":{\"max\":5,\"min\":0,\"tickInterval\":\"auto\"},\"internalTickHeightScaleFactor\":0.5,\"labelColor\":[255,255,200],\"labelFont\":{\"font\":\"Arial\",\"fontSize\":12},\"labelOffset\":0.05,\"labelTransparency\":1,\"needleImage\":{\"size\":[21,75],\"src\":\"data:image\\/svg+xml;base64,PHN2ZyB4bWxucz0iaHR0cDovL3d3dy53My5vcmcvMjAwMC9zdmciIHhtbG5zOnhsaW5rPSJodHRwOi8vd3d3LnczLm9yZy8xOTk5L3hsaW5rIiB2aWV3Qm94PSIwIDAgMjEgNzUiPjxkZWZzPjxzdHlsZT4uY2xzLTF7ZmlsbDpub25lO30uY2xzLTJ7aXNvbGF0aW9uOmlzb2xhdGU7fS5jbHMtM3tjbGlwLXBhdGg6dXJsKCNjbGlwLXBhdGgpO30uY2xzLTR7b3BhY2l0eTowLjM7bWl4LWJsZW5kLW1vZGU6bXVsdGlwbHk7fS5jbHMtNXtmaWxsOiNlYjI2Mjk7fTwvc3R5bGU+PGNsaXBQYXRoIGlkPSJjbGlwLXBhdGgiIHRyYW5zZm9y ...(+1928 chars)\",\"srcOrientation\":\"horizontal\"},\"needleOffset\":[0.007413509060955519,0],\"needleSize\":{\"height\":0.11955094537815127,\"width\":0.7589285714285714},\"position\":[0.015821953781512604,0.06944444444444445,0.7996031746031746,0.9641544117647058],\"referencePoint\":\"auto\",\"scaleColors\":[],\"scaleColorsSize\":0.2,\"scaleDirection\":\"BT\",\"showLabels\":1,\"showMinorTicks\":0,\"showSpanLine\":1,\"showTicks\":1,\"tickColor\":[252,252,197],\"tickTransparency\":1,\"valueBarColor\":[23,89,176],\"valueBarOffset\":0,\"valueBarSize\":0.23,\"valueBarTransparency\":1}},{\"name\":\"BackgroundImageComponent\",\"settings\":{\"image\":{\"size\":[380,101],\"src\":\"data:image\\/svg+xml;base64,PHN2ZyBpZD0iZnJhbWUiIHhtbG5zPSJodHRwOi8vd3d3LnczLm9yZy8yMDAwL3N2ZyIgeG1sbnM6eGxpbms9Imh0dHA6Ly93d3cudzMub3JnLzE5OTkveGxpbmsiIHZpZXdCb3g9IjAgMCAzODAgMTAxIj48ZGVmcz48c3R5bGU+LmNscy0xe2ZpbGw6IzAwMmI0Mjt9LmNscy0ye2ZpbGw6IzQyNzA4Mjt9LmNscy0ze2ZpbGw6dXJsKCNyYWRpYWwtZ3JhZGllbnQpO308L3N0eWxlPjxyYWRpYWxHcmFkaWVudCBpZD0icmFkaWFsLWdyYWRpZW50IiBjeD0iMTkwIiBjeT0iNTAuNSIgcj0iMjY5LjIxIiBncmFkaWVudFVuaXRzPSJ1c2VyU3BhY2VPblVzZSI+PHN0b3Agb2Zmc2V0PSIwLjAxIiBzdG9wLWNvbG9yPSIjM2U0ZjU4Ii8+PHN0b3Agb2Zmc2V0PSIwLjA2IiBzdG9wLWNvbG9yPSIjNDQ1NzYxIi8+PHN0b3Agb2Zmc2V0PSIwLjE1IiBzdG9wLWNvbG9yPSIjNTU2YTc2Ii8+PHN0b3Agb2Zmc2V0PSIwLjI1IiBzdG9wLWNvbG9yPSIjNmQ4ODk1Ii8+PHN0b3Agb2Zmc2V0PSIwLjM4IiBzdG9wLWNvbG9yPSIjOGZiMmMzIi8+PHN0b3Agb2Zmc2V0PSIwLjUyIiBzdG9wLWNvbG9yPSIjYjZlNGZhIi8+PHN0b3Agb2Zmc2V0PSIxIiBzdG9wLWNvbG9yPSIjMTU0NjU3Ii8+PC9yYWRpYWxHcmFkaWVudD48L2RlZnM+PGcgaWQ9IkxheWVyXzIiIGRhdGEtbmFtZT0iTGF5ZXIgMiI+PGcgaWQ9IkxheWVyXzEtMiIgZGF0YS1uYW1lPSJMYXllciAxLTIiPjxyZWN0IGlkPSJyZWN0MTAzNiIgY2xhc3M9ImNscy0xIiB4PSIxMSIgeT0iMTEiIHdpZHRoPSIzNTgiIGhlaWdodD0iNzkiLz48cGF0aCBpZD0icGF0aDEwMzgiIGNsYXNzPSJjbHMtMiIgZD0iTTgsOFY5M0gzNzJWOFpNMzY5LDkwSDExVjExSDM2OVoiLz48cGF0aCBpZD0icGF0aDEwNDAiIGNsYXNzPSJjbHMtMyIgZD0iTTAsMFYxMDFIMzgwVjBaTTM3Miw5M0g4VjhIMzcyWiIvPjwvZz48L2c+PC9zdmc+\",\"srcOrientation\":\"horizontal\"},\"position\":[0,0,1,1],\"scaleMode\":\"0\"}},{\"name\":\"ForegroundImageComponent\",\"settings\":{\"image\":{\"size\":[0,0],\"src\":\"default\",\"srcOrientation\":[]},\"isForeground\":1,\"position\":[0,0,1,1],\"scaleMode\":\"0\"}}],\"settings\":{\"BindingType\":\"signal\",\"backgroundColor\":[0,0,0,\"1\"],\"backgroundOffset\":0,\"backgroundOpacity\":1,\"fixedAspectRatio\":\"on\",\"orientation\":\"vertical\",\"showBackgroundColor\":false,\"value\":0,\"version\":\"R2023a\"},\"type\":\"LinearGauge\"}"

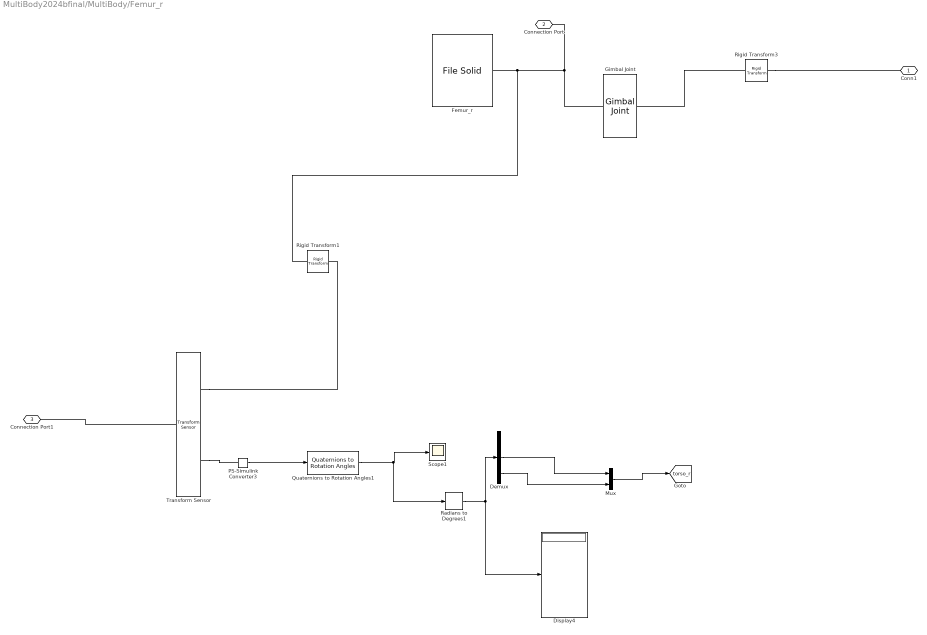
== system MultiBody2024bfinal/MultiBody/Femur_r ==
  Demux : Demux  Outputs=3
  Display4 : Display
  Femur_r : sm_lib/Body Elements/File Solid  ExtGeomFileName=D:\iit\iit\Cold Gas Thrusters\Supplementaries\Musculoskeletal full body model\obj\r_femur.obj  UnitType=Custom  ExtGeomFileUnits=m  StepReaderType=HEX  ExportConvexHullGeometry=off  InertiaType=Custom  BasedOnType=Mass  Density=1000  DensityUnits=kg/m^3  Mass=9.3013999999999992  MassUnits=kg  CenterOfMass=[0 -0.17000000000000001 0]  CenterOfMassUnits=m  MomentsOfInertia=[0.13389999999999999 0.035099999999999999 0.14119999999999999]  MomentsOfInertiaUnits=kg*m^2  ProductsOfInertia=[0 0 0]  ProductsOfInertiaUnits=kg*m^2  GraphicType=FromGeometry  MarkerShape=Sphere  MarkerSize=10  GraphicVisPropType=SimpleVisualProperties  GraphicDiffuseColor=[0.2 1.0 1.0]  GraphicOpacity=0.8  GraphicSpecularColor=[0.5 0.5 0.5 1.0]  GraphicAmbientColor=[0.15 0.15 0.15 1.0]  GraphicEmissiveColor=[0.0 0.0 0.0 1.0]  GraphicShininess=75  DoExposeReferenceFrame=on  SerializedFrames=<Frames/>
  Gimbal Joint : sm_lib/Joints/Gimbal Joint  JointMode=Normal  CompositeWrenchDir=FollowerOnBase  CompositeWrenchFrame=BaseFrame  SenseConstraintForce=off  SenseConstraintTorque=off  SenseTotalForce=off  SenseTotalTorque=off  RxPositionTargetSpecify=off  RxPositionTargetPriority=High  RxPositionTargetValue=-50  RxPositionTargetValueUnits=deg  RxVelocityTargetSpecify=off  RxVelocityTargetPriority=High  RxVelocityTargetValue=0  RxVelocityTargetValueUnits=deg/s  RxEquilibriumPosition=0  RxEquilibriumPositionUnits=deg  RxSpringStiffness=0  RxSpringStiffnessUnits=N*m/deg  RxDampingCoefficient=0  RxDampingCoefficientUnits=N*m/(deg/s)  RxLowerLimitSpecify=on  RxLowerLimitBound=-50  RxLowerLimitBoundUnits=deg  RxLowerLimitStiffness=1e4  RxLowerLimitStiffnessUnits=N*m/deg  RxLowerLimitDamping=10  RxLowerLimitDampingUnits=N*m/(deg/s)  RxLowerLimitTransitionRegionWidth=0.1  RxLowerLimitTransitionRegionWidthUnits=deg  RxUpperLimitSpecify=on  RxUpperLimitBound=30  RxUpperLimitBoundUnits=deg  RxUpperLimitStiffness=1e4  RxUpperLimitStiffnessUnits=N*m/deg  RxUpperLimitDamping=10  RxUpperLimitDampingUnits=N*m/(deg/s)  RxUpperLimitTransitionRegionWidth=0.1  RxUpperLimitTransitionRegionWidthUnits=deg  RxTorqueActuationMode=NoTorque  RxMotionActuationMode=ComputedMotion  RxSensePosition=off  RxSenseVelocity=off  RxSenseAcceleration=off  RxSenseTorqueForce=off  RxSenseLowerLimitTorqueForce=off  RxSenseUpperLimitTorqueForce=off  RyPositionTargetSpecify=off  RyPositionTargetPriority=High  RyPositionTargetValue=-40  RyPositionTargetValueUnits=deg  RyVelocityTargetSpecify=off  RyVelocityTargetPriority=High  RyVelocityTargetValue=0  RyVelocityTargetValueUnits=deg/s  RyEquilibriumPosition=0  RyEquilibriumPositionUnits=deg  RySpringStiffness=0  RySpringStiffnessUnits=N*m/deg  RyDampingCoefficient=0  RyDampingCoefficientUnits=N*m/(deg/s)  RyLowerLimitSpecify=on  RyLowerLimitBound=-40  RyLowerLimitBoundUnits=deg  RyLowerLimitStiffness=1e4  RyLowerLimitStiffnessUnits=N*m/deg  RyLowerLimitDamping=10  RyLowerLimitDampingUnits=N*m/(deg/s)  RyLowerLimitTransitionRegionWidth=0.1  RyLowerLimitTransitionRegionWidthUnits=deg  RyUpperLimitSpecify=on  RyUpperLimitBound=40  RyUpperLimitBoundUnits=deg  RyUpperLimitStiffness=1e4  RyUpperLimitStiffnessUnits=N*m/deg  RyUpperLimitDamping=10  RyUpperLimitDampingUnits=N*m/(deg/s)  RyUpperLimitTransitionRegionWidth=0.1  RyUpperLimitTransitionRegionWidthUnits=deg  RyTorqueActuationMode=NoTorque  RyMotionActuationMode=ComputedMotion  RySensePosition=off  RySenseVelocity=off  RySenseAcceleration=off  RySenseTorqueForce=off  RySenseLowerLimitTorqueForce=off  RySenseUpperLimitTorqueForce=off  RzPositionTargetSpecify=off  RzPositionTargetPriority=High  RzPositionTargetValue=-30  RzPositionTargetValueUnits=deg  RzVelocityTargetSpecify=off  RzVelocityTargetPriority=High  RzVelocityTargetValue=0  RzVelocityTargetValueUnits=deg/s  RzEquilibriumPosition=0  RzEquilibriumPositionUnits=deg  RzSpringStiffness=0  RzSpringStiffnessUnits=N*m/deg  RzDampingCoefficient=0  RzDampingCoefficientUnits=N*m/(deg/s)  RzLowerLimitSpecify=on  RzLowerLimitBound=-30  RzLowerLimitBoundUnits=deg  RzLowerLimitStiffness=1e4  RzLowerLimitStiffnessUnits=N*m/deg  RzLowerLimitDamping=10  RzLowerLimitDampingUnits=N*m/(deg/s)  RzLowerLimitTransitionRegionWidth=0.1  RzLowerLimitTransitionRegionWidthUnits=deg  RzUpperLimitSpecify=on  RzUpperLimitBound=120  RzUpperLimitBoundUnits=deg  RzUpperLimitStiffness=1e4  RzUpperLimitStiffnessUnits=N*m/deg  RzUpperLimitDamping=10  RzUpperLimitDampingUnits=N*m/(deg/s)  RzUpperLimitTransitionRegionWidth=0.1  RzUpperLimitTransitionRegionWidthUnits=deg  RzTorqueActuationMode=NoTorque  RzMotionActuationMode=ComputedMotion  RzSensePosition=off  RzSenseVelocity=off  RzSenseAcceleration=off  RzSenseTorqueForce=off  RzSenseLowerLimitTorqueForce=off  RzSenseUpperLimitTorqueForce=off
  Mux : Mux  Inputs=2
  PS-Simulink Converter3 : nesl_utility/PS-Simulink Converter  PhysicalDomain=network_engine_domain  SubClassName=ps_output  LeftPortType=input  RightPortType=output  PseudoPeriodic=off  Frequencies=[]  VectorFormat=inherit  Unit=inherit  AffineConversion=off
  Quaternions to Rotation Angles1 : sharedtransform/Quaternions to Rotation Angles  rotationOrder=ZYX  aMode=aMode
  Radians to Degrees1 : simulink_extras/Transformations/Radians to Degrees
  Rigid Transform1 : sm_lib/Frames and Transforms/Rigid Transform  RotationMethod=AlignedAxes  FollAlignAxisA=+X  BaseAlignAxisA=+X  FollAlignAxisB=+Z  BaseAlignAxisB=+Y  RotationStandardAxis=+Z  RotationAngle=0.0  RotationAngleUnits=deg  RotationArbitraryAxis=[0 0 1]  RotationSequenceAxes=FollowerAxes  RotationSequence=XYZ  RotationSequenceAngles=[-1.64157 1.44618 1.5708]  RotationSequenceAnglesUnits=rad  RotationMatrix=[1 0 0; 0 1 0; 0 0 1]  Quaternion=[1 0 0 0]  TranslationMethod=None  TranslationCartesianOffset=[-0.00809 -0.40795999999999999 -0.0027499999999999998]  TranslationCartesianOffsetUnits=m  TranslationStandardAxis=+X  TranslationStandardOffset=0.25  TranslationStandardOffsetUnits=m  TranslationROffset=0  TranslationROffsetUnits=m  TranslationThetaOffset=0  TranslationThetaOffsetUnits=deg  TranslationZOffset=0  TranslationZOffsetUnits=m
  Rigid Transform3 : sm_lib/Frames and Transforms/Rigid Transform  RotationMethod=None  FollAlignAxisA=+X  BaseAlignAxisA=+Y  FollAlignAxisB=+Y  BaseAlignAxisB=+Z  RotationStandardAxis=+Z  RotationAngle=0.0  RotationAngleUnits=deg  RotationArbitraryAxis=[0 0 1]  RotationSequenceAxes=FollowerAxes  RotationSequence=ZXY  RotationSequenceAngles=[90 0 0]  RotationSequenceAnglesUnits=deg  RotationMatrix=[1 0 0; 0 1 0; 0 0 1]  Quaternion=[1 0 0 0]  TranslationMethod=Cartesian  TranslationCartesianOffset=[-0.056276 -0.078490000000000004 0.0772599999999999950]  TranslationCartesianOffsetUnits=m  TranslationStandardAxis=+X  TranslationStandardOffset=0.25  TranslationStandardOffsetUnits=m  TranslationROffset=0  TranslationROffsetUnits=m  TranslationThetaOffset=0  TranslationThetaOffsetUnits=deg  TranslationZOffset=0  TranslationZOffsetUnits=m
  Scope1 : Scope
  Transform Sensor : sm_lib/Frames and Transforms/Transform Sensor  MeasurementFrame=NonRotatingBase  RotationSequence=XYZ  SenseAngle=off  SenseAxis=off  SenseQ=on  SenseR=off  SenseRotationSequence=off  SenseOmegaX=off  SenseOmegaY=off  SenseOmegaZ=off  SenseOmega=off  SenseQDot=off  SenseRDot=off  SenseRotationSequenceDot=off  SenseAlphaX=off  SenseAlphaY=off  SenseAlphaZ=off  SenseAlpha=off  SenseQDDot=off  SenseRDDot=off  SenseX=off  SenseY=off  SenseZ=off  SenseXYZ=off  SenseRad=off  SenseAzim=off  SenseDist=off  SenseInc=off  SenseXDot=off  SenseYDot=off  SenseZDot=off  SenseXYZDot=off  SenseRadDot=off  SenseAzimDot=off  SenseDistDot=off  SenseIncDot=off  SenseXDDot=off  SenseYDDot=off  SenseZDDot=off  SenseXYZDDot=off  SenseRadDDot=off  SenseAzimDDot=off  SenseDistDDot=off  SenseIncDDot=off
  Conn1 : PMIOPort  Side=Left
  Connection Port : PMIOPort  Port=2  Side=Left
  Connection Port1 : PMIOPort  Port=3  Side=Left
  tag scope: torso_r=global
  wires:
  Quaternions to Rotation Angles1/1 -> Radians to Degrees1/1, Scope1/1
  Radians to Degrees1/1 -> Demux/1, Display4/1
  PS-Simulink Converter3/1 -> Quaternions to Rotation Angles1/1
  Demux/3 -> Mux/2
  Mux/1 -> [torso_r]
  Demux/2 -> Mux/1
  connections:
  Rigid Transform3/RConn1 -- Gimbal Joint/LConn1
  Gimbal Joint/RConn1 -- Connection Port/RConn1 -- Rigid Transform1/RConn1 -- Femur_r/RConn1
  Rigid Transform3/LConn1 -- Conn1/RConn1
  Transform Sensor/RConn1 -- Rigid Transform1/LConn1
  Transform Sensor/RConn2 -- PS-Simulink Converter3/LConn1
  Transform Sensor/LConn1 -- Connection Port1/RConn1
